simulink model "msfcndemo_fi"  (Simulink 7.6)
settings: Solver=FixedStepDiscrete  StartTime=0.0  StopTime=10.0  RelTol=1e-3
settings Model: Creator=The MathWorks Inc.
settings OptimizationCC: EfficientMapNaN2IntZero=off

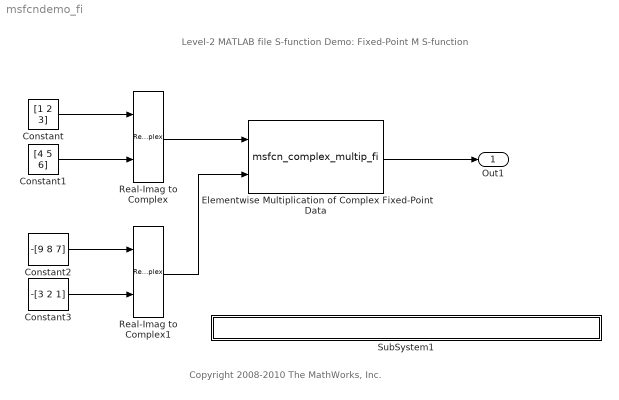
== system msfcndemo_fi ==
  note: Level-2 MATLAB file S-function Demo:
      | Fixed-Point M S-function
  note: Copyright 2008-2010 The MathWorks, Inc.
  Constant : Constant  Value=[1 2 3]  OutDataTypeStr=fixdt(1,16,2^-2,0)  SampleTime=.1
  Constant1 : Constant  Value=[4 5 6]  OutDataTypeStr=fixdt(1,16,2^-2,0)  SampleTime=.1
  Constant2 : Constant  Value=-[9 8 7]  OutDataTypeStr=fixdt(1,8,2^-2,0)  SampleTime=.1
  Constant3 : Constant  Value=-[3 2 1]  OutDataTypeStr=fixdt(1,8,2^-2,0)  SampleTime=.1
  Elementwise Multiplication of Complex Fixed-Point Data : M-S-Function  FunctionName=msfcn_complex_multip_fi
  Real-Imag to Complex : RealImagToComplex
  Real-Imag to Complex1 : RealImagToComplex
  SubSystem1 : Subsystem  mask{filename=msfcn_complex_multip_fi.m}
      mask init:
      | x=sfundemo_maskdisp;
      settings: AttributesFormatString=\n  OpenFcn=sfundemo_openfcn
      mask Display: disp(x);
  Out1 : Outport
  wires:
  Constant/1 -> Real-Imag to Complex/1
  Constant1/1 -> Real-Imag to Complex/2
  Elementwise Multiplication of Complex Fixed-Point Data/1 -> Out1/1
  Real-Imag to Complex/1 -> Elementwise Multiplication of Complex Fixed-Point Data/1
  Constant2/1 -> Real-Imag to Complex1/1
  Constant3/1 -> Real-Imag to Complex1/2
  Real-Imag to Complex1/1 -> Elementwise Multiplication of Complex Fixed-Point Data/2

== system msfcndemo_fi/SubSystem1 ==
